simulink model "SPMe_CC"  (R2022a)
settings: Solver=VariableStepAuto  StartTime=0.0  StopTime=t_end  MaxStep=1  RelTol=1e-6
values from neighbouring files (symbols this model uses):
  dt = 0.05    [run_SPMe_sweep.m]
  I = 4.6*C_rates(c)    [run_SPMe_sweep.m]
  ocv_init = 4.2    [run_SPMe_sweep.m]
  V_min = 0    [run_SPMe_sweep.m]
libraries: spsControlledCurrentSourceLib x1, spsControlledVoltageSourceLib x1, spsCurrentMeasurementLib x1, spsParallelRLCBranchLib x1, spspowerguiLib x1
settings Model: Creator=tom  LastModifiedBy=Vivian
settings SolverCC: AlgebraicLoopSolver=TrustRegion
settings DebuggingCC: UnconnectedInputMsg=warning  UnconnectedOutputMsg=warning  UnconnectedLineMsg=warning  SFMachineParentedDataDiag=warning
settings RTWCC: DLArmComputeVersion=19.05

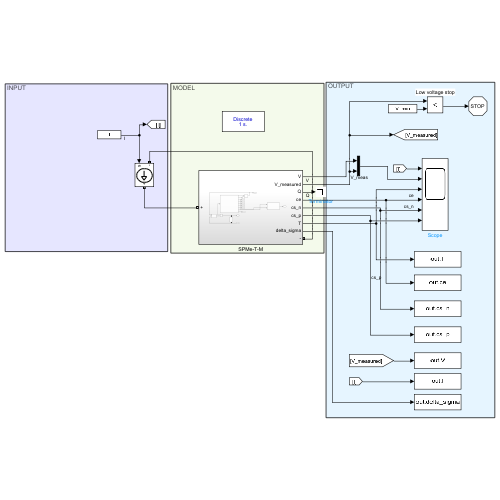
[thumbnail: Simulink's stored preview of the top-level diagram]
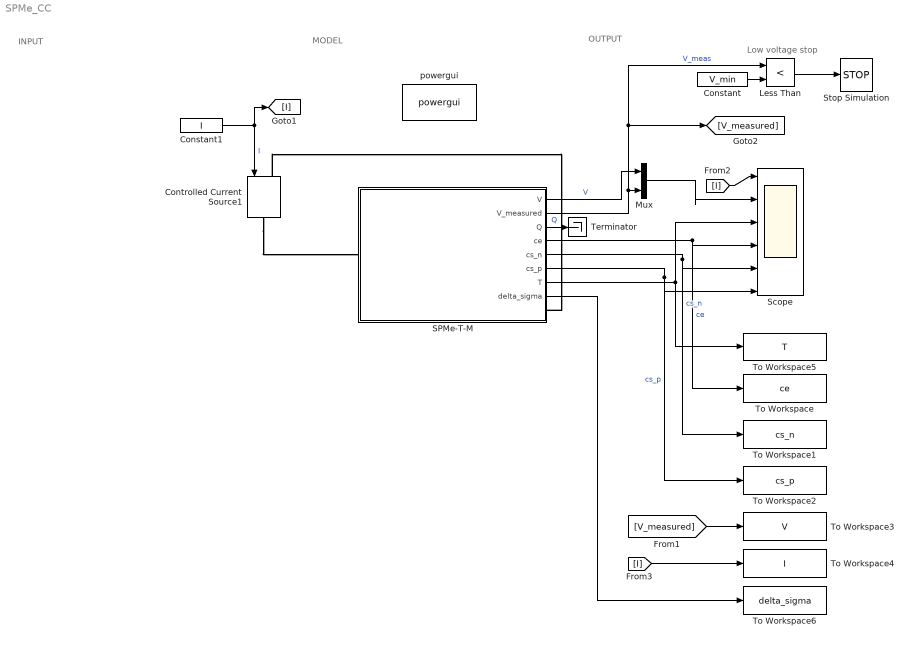
== system SPMe_CC ==
  note: OUTPUT
  note: MODEL
  note: INPUT
  note: Low voltage stop
  Constant : Constant  Value=V_min
  Constant1 : Constant  Value=I
  Controlled Current Source1 : spsControlledCurrentSourceLib/Controlled Current Source  Initialize=on  Source_Type=DC  Amplitude=0  Phase=0  Frequency=0  Measurements=None
  Less Than : RelationalOperator  Operator=<  OutDataTypeStr=boolean  RndMeth=Simplest  InputSameDT=off
  Mux : Mux  Inputs=2
  SPMe-T-M : Subsystem
  Scope : Scope  NumInputPorts=6
  Stop Simulation : Stop
  Terminator : Terminator
  To Workspace : ToWorkspace  VariableName=ce  SaveFormat=Timeseries  SampleTime=-1
  To Workspace1 : ToWorkspace  VariableName=cs_n  SaveFormat=Timeseries  SampleTime=-1
  To Workspace2 : ToWorkspace  VariableName=cs_p  SaveFormat=Timeseries  SampleTime=-1
  To Workspace3 : ToWorkspace  VariableName=V  SaveFormat=Timeseries  SampleTime=-1
  To Workspace4 : ToWorkspace  VariableName=I  SaveFormat=Timeseries  SampleTime=-1
  To Workspace5 : ToWorkspace  VariableName=T  SaveFormat=Timeseries  SampleTime=-1
  To Workspace6 : ToWorkspace  VariableName=delta_sigma  SaveFormat=Timeseries  SampleTime=-1
  powergui : spspowerguiLib/powergui  Priority=1  SimulationMode=Discrete  SampleTime=dt  frequency=60  Iterations=50  frequencyindice=0  Pbase=100e6  ErrMax=1e-4  UnitsV=kV  UnitsW=MW  buscounter=0  FunctionMessages=off  echomessages=off  EnableUseOfTLC=off  CurrentSourceSwitches=off  DisableSnubberDevices=off  DisableRonSwitches=off  DisableVfSwitches=off  DisplayEquations=off  AutomaticDiscreteSolvers=off  SolverType=Tustin/Backward Euler (TBE)  Interpol=off  ExternalGateDelay=off  methode=off  Ts=100  x0status=blocks  SPID=on  SwTol=0  HookPort=off  NonlinearTolerance=1e-4  nMaxIteration=100  ContinueOnMaxIteration=off  RestoreLinks=warning  ResistiveCurrentMeasurement=off  Frange=[0:2:500]  Ylog=off  Xlog=on  ShowGrid=off  save=off  variable=ZData  structure=0  ZoomFFT=off  StartTime=0.0  cycles=1  DisplayStyle=1  fundamental=60  FreqAxis=off  MaxFrequency=1000  frequencyindicesteady=1  RmsSteady=1  display=off
  wires:
  SPMe-T-M/5(cs_n) -> To Workspace1/1, Scope/5  "cs_n"
  SPMe-T-M/6(cs_p) -> To Workspace2/1, Scope/6  "cs_p"
  Less Than/1 -> Stop Simulation/1
  Constant/1 -> Less Than/2
  SPMe-T-M/4(ce) -> To Workspace/1, Scope/4  "ce"
  SPMe-T-M/1(V) -> Mux/1  "V"
  SPMe-T-M/2(V_measured) -> Less Than/1, [V_measured], Mux/2  "V_meas"
  Constant1/1 -> Controlled Current Source1/1, [I]  "I"
  Mux/1 -> Scope/2
  [V_measured] -> To Workspace3/1
  [I] -> Scope/1
  [I] -> To Workspace4/1
  SPMe-T-M/8(delta_sigma) -> To Workspace6/1
  SPMe-T-M/3(Q) -> Terminator/1  "Q"
  SPMe-T-M/7(T) -> To Workspace5/1, Scope/3
  connections:
  Controlled Current Source1/RConn1 -- SPMe-T-M/LConn1
  Controlled Current Source1/LConn1 -- SPMe-T-M/RConn1

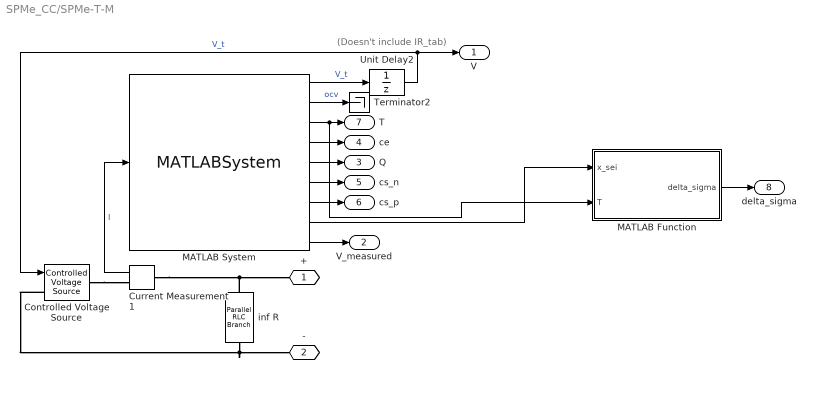
== system SPMe_CC/SPMe-T-M ==
  note: (Doesn't include IR_tab)
  Controlled Voltage Source : spsControlledVoltageSourceLib/Controlled Voltage Source  Initialize=on  Source_Type=AC  Amplitude=0  Phase=0  Frequency=0  Measurements=None
  Current Measurement1 : spsCurrentMeasurementLib/Current Measurement  PhasorSimulation=off  OutputType=Complex  PSBequivalent=0
  MATLAB Function : MATLAB Function  TreatAsAtomicUnit=on
  MATLAB System : MATLABSystem  System=pybamm_bat  SimulateUsing=Interpreted execution
      mask Type: pybamm_bat
      mask Display:
      | disp('pybamm_bat');
      | port_label('input',1,'current');
      | port_label('output',1,'V_t');
      | port_label('output',2,'ocv');
      | port_label('output',3,'T');
      | port_label('output',4,'ce');
      | port_label('output',5,'heating');
      | port_label('output',6,'neg_conc');
      | port_label('output',7,'pos_conc');
      | port_label('output',8,'x_sei');
      | port_label('output',9,'V_meas');
  Terminator2 : Terminator
  Unit Delay2 : UnitDelay  InitialCondition=ocv_init  SampleTime=-1  HasFrameUpgradeWarning=on
  inf R : spsParallelRLCBranchLib/Parallel RLC Branch  LConnTagsString=a  RConnTagsString=__new0  BranchType=R  Resistance=1e8  Inductance=1e-3  SetiL0=off  InitialCurrent=0  Capacitance=1e-6  Setx0=off  InitialVoltage=0  Measurements=None
  + : PMIOPort  Tag=PMCPort  Side=Left
  - : PMIOPort  Tag=PMCPort  Port=2  Side=Right
  V : Outport
  V_measured : Outport  Port=2
  Q : Outport  Port=3  VectorParamsAs1DForOutWhenUnconnected=off
  ce : Outport  Port=4
  cs_n : Outport  Port=5  VectorParamsAs1DForOutWhenUnconnected=off
  cs_p : Outport  Port=6  VectorParamsAs1DForOutWhenUnconnected=off
  T : Outport  Port=7
  delta_sigma : Outport  Port=8
  wires:
  Current Measurement1/1 -> MATLAB System/1  "I"
  MATLAB System/4 -> ce/1
  MATLAB System/5 -> Q/1
  MATLAB System/6 -> cs_n/1
  MATLAB System/7 -> cs_p/1
  MATLAB System/1 -> Unit Delay2/1  "V_t"
  Unit Delay2/1 -> V/1, Controlled Voltage Source/1  "V_t"
  MATLAB System/8 -> MATLAB Function/1(x_sei)
  MATLAB System/9 -> V_measured/1
  MATLAB System/3 -> MATLAB Function/2(T), T/1
  MATLAB System/2 -> Terminator2/1  "ocv"
  MATLAB Function/1(delta_sigma) -> delta_sigma/1
  connections:
  inf R/LConn1 -- +/RConn1 -- Current Measurement1/LConn1
  inf R/RConn1 -- Controlled Voltage Source/LConn1 -- -/RConn1
  Controlled Voltage Source/RConn1 -- Current Measurement1/RConn1

== matlab function SPMe_CC/SPMe-T-M/MATLAB Function ==
  data: x_sei input; delta_sigma output; T input
function delta_sigma  = expansion(x_sei, T)
%XSEI2PTOTAL 
% Mechanical params
M_C6 = 72/1000; %kg/mol
% V_head_0 = 6.65e-6; %m3 (0.121*0.074*0.0055)*0.135
% L = 2.4/1000; %m
% E = 0.19e6; %Pa
% alpha_cell = 1.1e-6; %m/K
% P_atm = 101; %kPa
% P_crit = 158.7731; %kPa
R = 8.3145; %J.mol-1.K-1
A = 0.009; %m2 (0.121*0.074)
DMC = [6.4338; 1413; -44.25]; %Antoine coeffs [A B C] 
EC = [6.4897; 1836.57; -102.23];
y_dmc = 0.7;
y_ec = 1-y_dmc;         
m_an = 0.0191; 
x_sei_0 = 0.15;
% T_amb = 273.15+25; % K
% sigma_0 = 1.5120e+04;

% Internal cell pressure
V_head_0 = 6.65e-06; %m-3
L_p0 = 2.4e-3; %m for 2 poron
E_p = 0.19e6; %Pa Young's modulus for poron
% E_c = 1e12; %assume large by default
alpha = 1.1e-6; %m/K
P_atm = 101e3; %Pa
% P_crit = 158e3; %Pa
% P0 = 14e3; %Pa
R = 8.3145; %J.mol-1.K-1
% k_b = 1.380649e-23; %m2.kg.s-2.K-1;
T_amb = 273.15+25; % K
sigma_0 = 1.5120e+04;
% L_cs0 = 5.5e-3; %m initial cell solid thickness
% V_cell = 0.130*0.089*0.055; % [130mm×89mm×5.5mm] active material

% P_elyte
Psat_EC = 10.^(EC(1)-EC(2)./(EC(3)+T));
Psat_DMC = 10.^(DMC(1)-DMC(2)./(DMC(3)+T)); 
P_elyte = (y_dmc*Psat_DMC + y_ec*Psat_EC)*1e3; 

% P_CO2
n_CO2 = 0.5*m_an/M_C6*(x_sei_0-x_sei);

% Solve for gas volume and pressure
delta_sigma_calc = P_elyte - sigma_0 - P_atm;
a = 1;
b = -(V_head_0 + A.*(L_p0/E_p*(delta_sigma_calc) - alpha.*(T-T_amb)));
c = -A*L_p0/E_p.*n_CO2.*R.*(T);
V_g0 = (-b+sqrt(max(b.^2-4.*a.*c,0)))/(2*a);
V_g = max(V_g0, V_head_0); % min V_g = V_head_0

P_CO2 = n_CO2.*R.*T./V_g;
P_gas = P_elyte + P_CO2;

delta_sigma = max(P_gas-P_atm-sigma_0, E_p./L_p0.*alpha.*(T-T_amb));
end
